simulink model "validacion_subsistema_electromagnetico"  (R2023b)
settings: Solver=VariableStepAuto  StartTime=0.0  StopTime=10.0  RelTol=1e-3
values from neighbouring files (symbols this model uses):
  alpha_Cu = 3.9e-3    (= 0.0039)    [controlador_foc_simulink.m]    (also in parametros_planta.m; params_subsistema_electromagnetico.m; params_subsistema_termico.m; sistema_completo_en_codigo.m)
  L_d = 6.6e-3    (= 0.0066)    [controlador_foc_simulink.m]    (also in params_subsistema_electromagnetico.m; sistema_completo_en_codigo.m)
  L_l = 0.8e-3    (= 0.0008)    [controlador_foc_simulink.m]    (also in params_subsistema_electromagnetico.m; sistema_completo_en_codigo.m)
  L_q = 5.8e-3    (= 0.0058)    [controlador_foc_simulink.m]    (also in params_subsistema_electromagnetico.m; sistema_completo_en_codigo.m)
  lambda_m = 0.016    [controlador_foc_simulink.m]    (also in parametros_planta.m; params_subsistema_electromagnetico.m; sistema_completo_en_codigo.m)
  Pp = 3    [controlador_foc_simulink.m]    (also in parametros_planta.m; params_subsistema_electromagnetico.m; sistema_completo_en_codigo.m)
  Rs_REF = 1.02    [controlador_foc_simulink.m]    (also in parametros_planta.m; params_subsistema_electromagnetico.m; params_subsistema_termico.m; sistema_completo_en_codigo.m)
  T_s_test = 40    [plot_validacion_subsistema_electromagnetico.m]
  theta_m_test = 0    [plot_validacion_subsistema_electromagnetico.m]
  Ts_REF = 20.0    (= 20)    [controlador_foc_simulink.m]    (also in parametros_planta.m; params_subsistema_electromagnetico.m; params_subsistema_termico.m; sistema_completo_en_codigo.m)
  va_amp = 0    [plot_validacion_subsistema_electromagnetico.m]
  vb_amp = 10 * (sqrt(3)/2)    [plot_validacion_subsistema_electromagnetico.m]
  vc_amp = -10 * (sqrt(3)/2)    [plot_validacion_subsistema_electromagnetico.m]
  w_m_test = 0    [plot_validacion_subsistema_electromagnetico.m]
libraries: eeTransforms x2
settings Model: Creator=Pc  LastModifiedBy=Pc

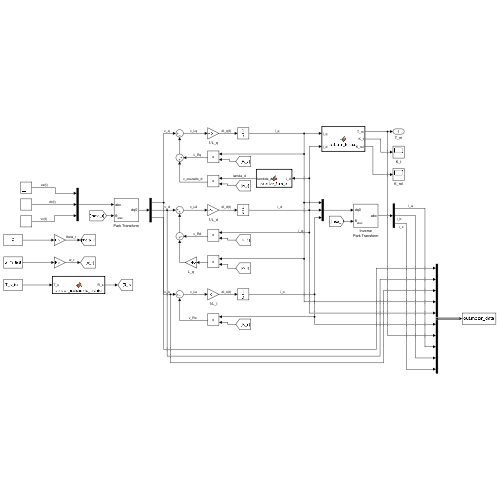
[thumbnail: Simulink's stored preview of the top-level diagram]
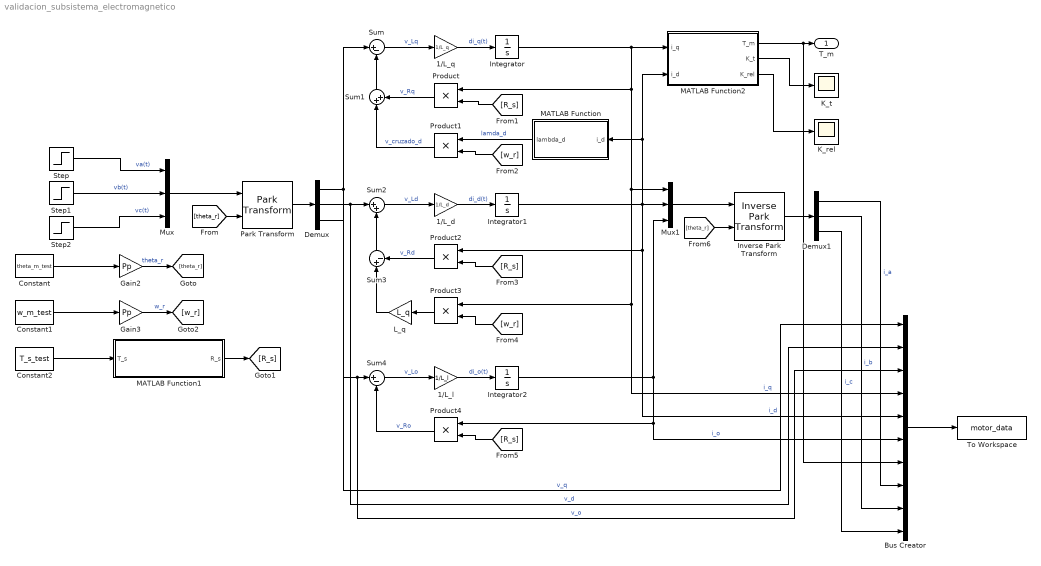
== system validacion_subsistema_electromagnetico ==
  1/L_d : Gain  Gain=1/L_d
  1/L_l : Gain  Gain=1/L_l
  1/L_q : Gain  Gain=1/L_q
  Bus Creator : BusCreator  Inputs=10
  Constant : Constant  Value=theta_m_test
  Constant1 : Constant  Value=w_m_test
  Constant2 : Constant  Value=T_s_test
  Demux : Demux  Outputs=3
  Demux1 : Demux  Outputs=3
  Gain2 : Gain  Gain=Pp
  Gain3 : Gain  Gain=Pp
  Integrator : Integrator
  Integrator1 : Integrator
  Integrator2 : Integrator
  Inverse Park Transform : eeTransforms/Inverse Park Transform  AxisAlignment=Q-axis  PowerInvariant=off
      settings: LibrarySourceBlock=|
      | ee_sl_lib/Mathematical
      | Transforms/Inverse
      | Park Transform
  K_rel : Scope
  K_t : Scope
  L_q : Gain  Gain=L_q
  MATLAB Function : MATLAB Function  TreatAsAtomicUnit=on
  MATLAB Function1 : MATLAB Function  TreatAsAtomicUnit=on
  MATLAB Function2 : MATLAB Function  TreatAsAtomicUnit=on
  Mux : Mux  Inputs=3
  Mux1 : Mux  Inputs=3
  Park Transform : eeTransforms/Park Transform  AxisAlignment=Q-axis  PowerInvariant=off
      settings: LibrarySourceBlock=|
      | ee_sl_lib/Mathematical
      | Transforms/Park Transform
  Product{,1..4} (5 alike) : Product
  Step : Step  After=va_amp  SampleTime=0
  Step1 : Step  After=vb_amp  SampleTime=0
  Step2 : Step  After=vc_amp  SampleTime=0
  Sum : Sum  Inputs=|+-
  Sum1 : Sum  Inputs=|++
  Sum2 : Sum  Inputs=|++
  Sum3 : Sum  Inputs=|+-
  Sum4 : Sum  Inputs=|+-
  To Workspace : ToWorkspace  VariableName=motor_data  SaveFormat=Timeseries  SampleTime=-1
  T_m : Outport
  wires:
  Mux/1 -> Park Transform/1
  Step1/1 -> Mux/2  "vb(t)"
  Step2/1 -> Mux/3  "vc(t)"
  Step/1 -> Mux/1  "va(t)"
  [theta_r] -> Park Transform/2
  Park Transform/1 -> Demux/1
  Integrator/1 -> Product/1, Mux1/1, Bus Creator/4, Product3/1, MATLAB Function2/1(i_q)  "i_q"
  1/L_q/1 -> Integrator/1  "di_q(t)"
  Demux/1 -> Bus Creator/1, Sum/1  "v_q"
  Sum1/1 -> Sum/2
  Sum/1 -> 1/L_q/1  "v_Lq"
  Product/1 -> Sum1/2  "v_Rq"
  [R_s] -> Product/2
  MATLAB Function/1(lambda_d) -> Product1/1  "lamda_d"
  Product1/1 -> Sum1/1  "v_cruzado_d"
  Constant/1 -> Gain2/1
  Gain2/1 -> [theta_r]  "theta_r"
  Constant1/1 -> Gain3/1
  Gain3/1 -> [w_r]  "w_r"
  [w_r] -> Product1/2
  1/L_d/1 -> Integrator1/1  "di_d(t)"
  Sum3/1 -> Sum2/2
  Demux/2 -> Sum2/1, Bus Creator/2  "v_d"
  Sum2/1 -> 1/L_d/1  "v_Ld"
  Integrator1/1 -> Product2/1, Bus Creator/5, MATLAB Function/1(i_d), MATLAB Function2/2(i_d), Mux1/2  "i_d"
  Product2/1 -> Sum3/2  "v_Rd"
  [R_s] -> Product2/2
  [w_r] -> Product3/2
  Product3/1 -> L_q/1
  L_q/1 -> Sum3/1
  1/L_l/1 -> Integrator2/1  "di_o(t)"
  Sum4/1 -> 1/L_l/1  "v_Lo"
  Demux/3 -> Bus Creator/3, Sum4/1  "v_o"
  [R_s] -> Product4/2
  Product4/1 -> Sum4/2  "v_Ro"
  Integrator2/1 -> Product4/1, Bus Creator/6, Mux1/3  "i_o"
  Mux1/1 -> Inverse Park Transform/1
  [theta_r] -> Inverse Park Transform/2
  Inverse Park Transform/1 -> Demux1/1
  Demux1/1 -> Bus Creator/8  "i_a"
  Demux1/2 -> Bus Creator/9  "i_b"
  Demux1/3 -> Bus Creator/10  "i_c"
  Constant2/1 -> MATLAB Function1/1(T_s)
  MATLAB Function1/1(R_s) -> [R_s]
  MATLAB Function2/1(T_m) -> Bus Creator/7, T_m/1
  MATLAB Function2/2(K_t) -> K_t/1
  MATLAB Function2/3(K_rel) -> K_rel/1
  Bus Creator/1 -> To Workspace/1

== matlab function validacion_subsistema_electromagnetico/MATLAB Function1 ==
  data: T_s input; R_s output; Rs_REF parameter; Ts_REF parameter; alpha_Cu parameter
function R_s = calcular_resistencia_estator(T_s, Rs_REF, Ts_REF, alpha_Cu)
    % CALCULAR_RESISTENCIA_ESTATOR Calcula la resistencia dinámica del estator
    % en función de su temperatura actual.
    %
    % Entradas:
    %   T_s      : Temperatura instantánea del estator [°C] (Señal dinámica Inport).
    %   Rs_REF   : Resistencia nominal de referencia [Ohm] (Parámetro).
    %   Ts_REF   : Temperatura nominal de referencia [°C] (Parámetro).
    %   alpha_Cu : Coeficiente de temperatura del cobre [1/°C] (Parámetro).
    %
    % Salida:
    %   R_s      : Resistencia actual del estator [Ohm].

    % Cálculo lineal de la resistencia por temperatura
    R_s = Rs_REF * (1 + alpha_Cu * (T_s - Ts_REF));
end

== matlab function validacion_subsistema_electromagnetico/MATLAB Function ==
  data: i_d input; lambda_d output; lambda_m parameter; L_d parameter
function lambda_d = calcular_flujo_d(i_d, lambda_m, L_d)
    % CALCULAR_FLUJO_D Calcula el flujo magnético total concatenado en el eje directo (d).
    %
    % Entradas:
    %   i_d      : Corriente instantánea en el eje d (Señal dinámica de entrada).
    %   lambda_m : Flujo de los imanes permanentes (Parámetro estático).
    %   L_d      : Inductancia del estator en el eje d (Parámetro estático).
    %
    % Salida:
    %   lambda_d : Flujo magnético total en el eje d.

    % Cálculo: Flujo de imanes + Flujo de reacción del inducido
    lambda_d = lambda_m + L_d * i_d;
end

== matlab function validacion_subsistema_electromagnetico/MATLAB Function2 ==
  data: i_q input; i_d input; T_m output; Pp parameter; lambda_m parameter; L_d parameter; L_q parameter; K_t output; K_rel output
function [T_m, K_t, K_rel] = calcular_torque(i_q, i_d, Pp, lambda_m, L_d, L_q)
    % CALCULAR_TORQUE Calcula el torque electromagnético total de la máquina PMSM
    % y sus constantes equivalentes.
    % 
    % Entradas dinámicas (Inports):
    %   i_q      : Corriente en el eje en cuadratura [A].
    %   i_d      : Corriente en el eje directo [A].
    %
    % Parámetros estáticos (Parameters):
    %   P_p      : Número de pares de polos.
    %   lambda_m : Flujo magnético de los imanes permanentes [Wb].
    %   L_d      : Inductancia del eje d [H].
    %   L_q      : Inductancia del eje q [H].
    %
    % Salidas:
    %   T_m      : Torque electromagnético generado [N.m].
    %   K_t      : Constante de torque de alineación [N.m/A].
    %   K_rel    : Constante de torque de reluctancia [N.m/A^2].

    % 1. Cálculo de las constantes 
    K_t = (3/2) * Pp * lambda_m;
    K_rel = (3/2) * Pp * (L_d - L_q);

    % 2. Cálculo del torque electromagnético total
    T_m = K_t * i_q + K_rel * i_d * i_q;
end
